simulink model "Matrix_product"  (Simulink 8.0)
settings: Solver=ode45  StartTime=0.0  StopTime=10.0  RelTol=1e-3
settings Model: Creator=Faradars  LastModifiedBy=Faradars

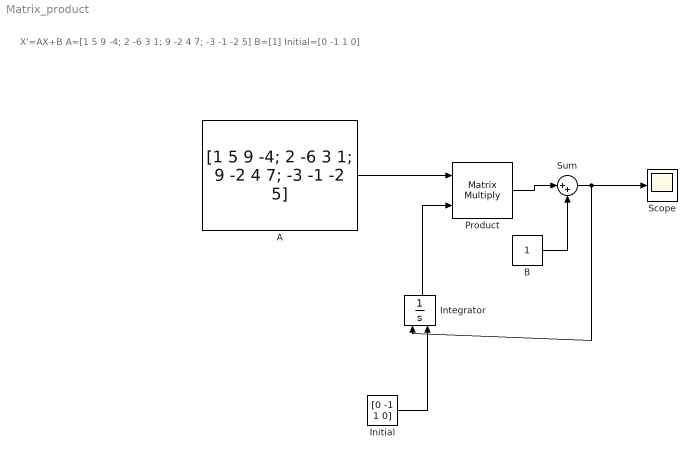
== system Matrix_product ==
  note: X'=AX+B
      | A=[1 5 9 -4; 2 -6 3 1; 9 -2 4 7; -3 -1 -2 5]
      | B=[1]
      | Initial=[0 -1 1 0]
  A : Constant  Value=[1 5 9 -4; 2 -6 3 1; 9 -2 4 7; -3 -1 -2 5]
  B : Constant
  Initial : Constant  Value=[0 -1 1 0]
  Integrator : Integrator  InitialConditionSource=external
  Product : Product  Multiplication=Matrix(*)  RndMeth=Zero
  Scope : Scope
  Sum : Sum  Inputs=|++
  wires:
  A/1 -> Product/1
  Product/1 -> Sum/1
  B/1 -> Sum/2
  Sum/1 -> Scope/1, Integrator/1
  Integrator/1 -> Product/2
  Initial/1 -> Integrator/2
